simulink model "PCM_SIM"  (R2024a)
settings: Solver=VariableStepAuto  StartTime=0.0  StopTime=10.0  RelTol=1e-3
libraries: dspquant2 x2, dspfdesign x1
settings Model: Creator=adity  LastModifiedBy=adity

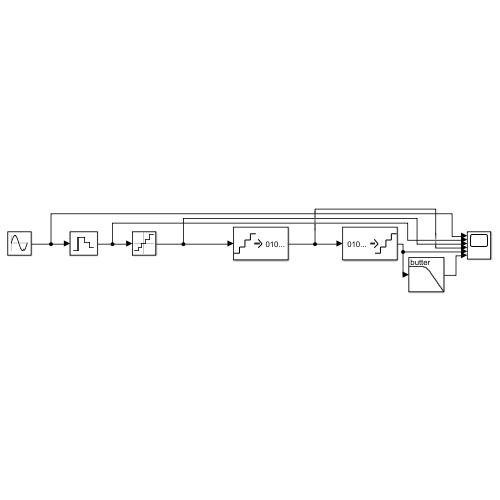
[thumbnail: Simulink's stored preview of the top-level diagram]
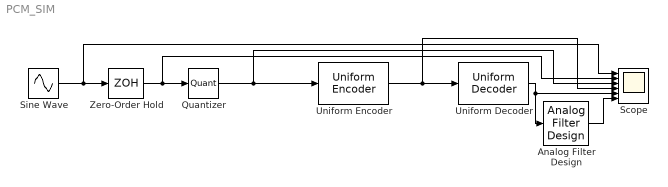
== system PCM_SIM ==
  Analog Filter Design : dspfdesign/Analog Filter Design  method=Butterworth  filttype=Lowpass  N=2  Wlo=5  Whi=80  Rp=2  Rs=40
  Quantizer : Quantizer  QuantizationInterval=0.1
  Scope : Scope  NumInputPorts=6
  Sine Wave : Sin  SampleTime=0
  Uniform Decoder : dspquant2/Uniform Decoder  peak=1  bits=8  overflowMode=Saturate  otype=double
  Uniform Encoder : dspquant2/Uniform Encoder  peak=1  bits=8  otype=Unsigned integer
  Zero-Order Hold : ZeroOrderHold  SampleTime=-1
  wires:
  Sine Wave/1 -> Scope/1, Zero-Order Hold/1
  Zero-Order Hold/1 -> Scope/2, Quantizer/1
  Quantizer/1 -> Scope/3, Uniform Encoder/1
  Uniform Encoder/1 -> Scope/4, Uniform Decoder/1
  Uniform Decoder/1 -> Analog Filter Design/1, Scope/5
  Analog Filter Design/1 -> Scope/6
